simulink model "AFE_FV_RC_2L_Hacheur_4_Quadrants"  (R2013a)
settings: Solver=FixedStepDiscrete  SolverMode=SingleTasking  StartTime=0.0  StopTime=inf  FixedStep=Tpas  RelTol=1e-3
values from neighbouring files (symbols this model uses):
  Cbus = 300e-3    (= 0.3)    [AFE_FV_Params.m]
  Freq = 50    [AFE_FV_Params.m]
  hys = 100    [AFE_FV_Params.m]
  Iv = (Pv+Numdv(2)/Dendv(1))/Tsv    [AFE_FV_Params.m]
  Kac = 1/(Vac*sqrt(2/3))    [AFE_FV_Params.m]
  Lac = 8.1487e-04    (= 0.00081487)    [AFE_FV_Params.m]
  Pv = Numdv(1)/Dendv(1)    [AFE_FV_Params.m]
  Rch = 12    [AFE_FV_Params.m]
  Satv = 1500    [AFE_FV_Params.m]
  Tpas = 5e-5    (= 5e-05)    [AFE_FV_Params.m]
  Vac = 2000    [AFE_FV_Params.m]
undefined symbols (not defined in the file or in its folder): Rac
libraries: powerlib x30, simulink x8, powerlib_meascontrol x7
settings Model: Creator=LiberT  LastModifiedBy=Francis
settings DataIOCC: SignalLoggingSaveFormat=ModelDataLogs
settings OptimizationCC: ExpressionDepthLimit=2147483647
settings DebuggingCC: MultiTaskDSMMsg=warning  MultiTaskCondExecSysMsg=none  FcnCallInpInsideContextMsg=EnableAllAsWarning  StrictBusMsg=None
settings RTWCC: IncludeERTFirstTime=on

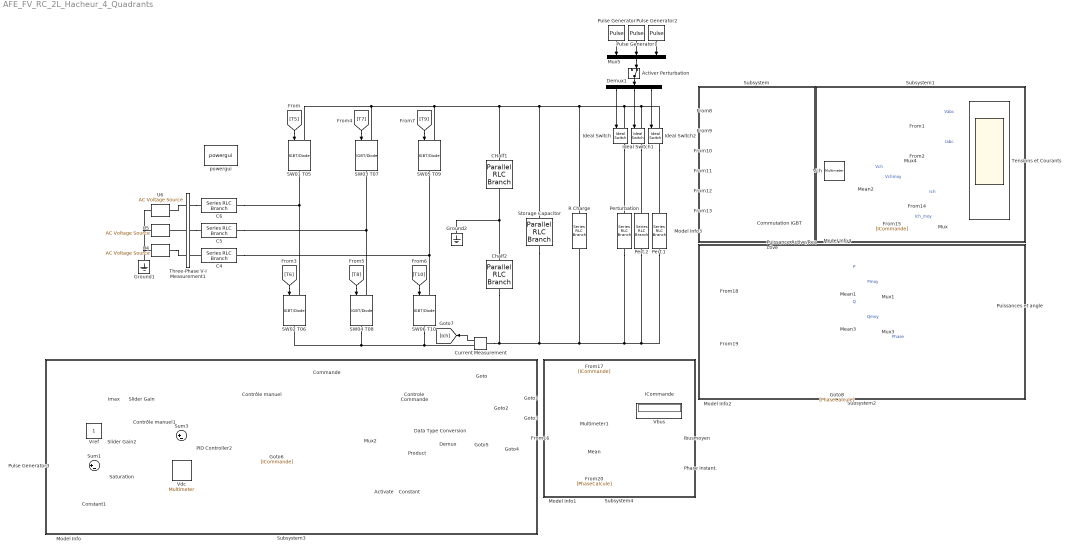
== system AFE_FV_RC_2L_Hacheur_4_Quadrants ==
  Activate : Constant  Value=0
  Activer Perturbation : ManualSwitch  CurrentSetting=0
  C4 : powerlib/Elements/Series RLC Branch  LConnTagsString=__new0  RConnTagsString=__new0  BranchType=L  Resistance=Rac  Inductance=Lac  SetiL0=off  InitialCurrent=0  Capacitance=300e-3  Setx0=off  InitialVoltage=0  Measurements=None
  C5 : powerlib/Elements/Series RLC Branch  LConnTagsString=__new0  RConnTagsString=__new0  BranchType=L  Resistance=Rac  Inductance=Lac  SetiL0=off  InitialCurrent=0  Capacitance=300e-3  Setx0=off  InitialVoltage=0  Measurements=None
  C6 : powerlib/Elements/Series RLC Branch  LConnTagsString=__new0  RConnTagsString=__new0  BranchType=L  Resistance=Rac  Inductance=Lac  SetiL0=off  InitialCurrent=0  Capacitance=300e-3  Setx0=off  InitialVoltage=0  Measurements=None
  CHalf1 : powerlib/Elements/Parallel RLC Branch  LConnTagsString=a  RConnTagsString=__new0  BranchType=C  Resistance=inf  Inductance=inf  SetiL0=off  InitialCurrent=0  Capacitance=.018  Setx0=off  InitialVoltage=2500  Measurements=Branch voltage
  Chalf2 : powerlib/Elements/Parallel RLC Branch  LConnTagsString=a  RConnTagsString=__new0  BranchType=C  Resistance=inf  Inductance=inf  SetiL0=off  InitialCurrent=0  Capacitance=.018  Setx0=off  InitialVoltage=2500  Measurements=Branch voltage
  Commande : Subsystem
  Commutation IGBT : Scope  NumInputPorts=6
      settings: TickLabels=on  TimeRange=0.04  YMin=-0.2~-0.2~-0.2~-0.2~-0.2~-0.2  YMax=1.2~1.2~1.2~1.2~1.2~1.2
  Constant : Constant  Value=[1 1 1 1 1 1]
  Constant1 : Constant  Value=6000
  Controle Commande : ManualSwitch
  Contrôle manuel : ManualSwitch  CurrentSetting=0
  Contrôle manuel1 : ManualSwitch  CurrentSetting=0
  Current Measurement : powerlib/Measurements/Current Measurement  PhasorSimulation=off  OutputType=Complex  PSBequivalent=0
  Data Type Conversion : DataTypeConversion  OutDataTypeStr=boolean
  Demux : Demux  Outputs=6
  Demux1 : Demux  Outputs=3
  Ground1 : powerlib/Elements/Ground  LConnTagsString=a
  Ground2 : powerlib/Elements/Ground  LConnTagsString=a
  "ICommande " : Display
  Ibusmoyen : Display
  Ideal Switch : powerlib/Power Electronics/Ideal Switch  Ron=0.001  Lon=0  IC=0  Rs=1e5  Cs=inf  Measurements=on
  Ideal Switch1 : powerlib/Power Electronics/Ideal Switch  Ron=0.001  Lon=0  IC=0  Rs=1e5  Cs=inf  Measurements=on
  Ideal Switch2 : powerlib/Power Electronics/Ideal Switch  Ron=0.001  Lon=0  IC=0  Rs=1e5  Cs=inf  Measurements=on
  Imax : Constant  Value=5000
  Mean{,1..3} (4 alike) : powerlib_meascontrol/Measurements/Mean  Freq=50  Vinit=0  Ts=Tpas
  Model Info : simulink/Model-Wide Utilities/Model Info  InitialBlockCM=None  BlockCM=None  Frame=on  DisplayStringWithTags=Commande  HorizontalTextAlignment=Center  LeftAlignmentValue=0.5  SourceBlockDiagram=AFE_FV_RC_2L_Hys  TagMaxNumber=20
  Model Info{1..4} (4 alike) : simulink/Model-Wide Utilities/Model Info  InitialBlockCM=None  BlockCM=None  Frame=on  DisplayStringWithTags=Résultats  HorizontalTextAlignment=Center  LeftAlignmentValue=0.5  SourceBlockDiagram=AFE_FV_RC_2L_Hys  TagMaxNumber=20
  Multimeter1 : powerlib/Measurements/Multimeter  PhasorSimulation=off  OutputType=Complex  sel=1  L=6  Gain=1  yselected={'Ub: Storage Capacitor'};  PSBOutputType=1  PSBequivalent=0  AxesSetting=[0,0.1,-100,100]  Display=0  SavedBlockNames=-11
  Mux{,1,3..4} (4 alike) : Mux  Inputs=2
  Mux2 : Mux  Inputs=6
  Mux5 : Mux  Inputs=3
  PID Controller2 : simulink/Continuous/PID Controller  Controller=PI  TimeDomain=Discrete-time  SampleTime=Tpas  IntegratorMethod=Forward Euler  FilterMethod=Forward Euler  Form=Parallel  P=Pv  I=Iv  D=0  N=100  InitialConditionSource=internal  InitialConditionForIntegrator=0  InitialConditionForFilter=0  ExternalReset=none  LimitOutput=on  UpperSaturationLimit=Satv  LowerSaturationLimit=-Satv  LinearizeAsGain=on  AntiWindupMode=clamping  Kb=1  TrackingMode=off  Kt=1  PParamMin=[]  PParamMax=[]  IParamMin=[]  IParamMax=[]  DParamMin=[]  DParamMax=[]  NParamMin=[]  NParamMax=[]  KbParamMin=[]  KbParamMax=[]  KtParamMin=[]  KtParamMax=[]  POutMin=[]  POutMax=[]  IOutMin=[]  IOutMax=[]  DOutMin=[]  DOutMax=[]  NOutMin=[]  NOutMax=[]  KbOutMin=[]  KbOutMax=[]  KtOutMin=[]  KtOutMax=[]  IntegratorOutMin=[]  IntegratorOutMax=[]  FilterOutMin=[]  FilterOutMax=[]  SumOutMin=[]  SumOutMax=[]  SumI1OutMin=[]  SumI1OutMax=[]  SumI2OutMin=[]  SumI2OutMax=[]  SumI3OutMin=[]  SumI3OutMax=[]  SumDOutMin=[]  SumDOutMax=[]  SaturationOutMin=[]  SaturationOutMax=[]  IntegratorContinuousStateAttributes=''  IntegratorStateMustResolveToSignalObject=off  IntegratorRTWStateStorageClass=Auto  FilterContinuousStateAttributes=''  FilterStateMustResolveToSignalObject=off  FilterRTWStateStorageClass=Auto
  Pert.1 : powerlib/Elements/Series RLC Branch  LConnTagsString=__new0  RConnTagsString=__new0  BranchType=R  Resistance=50  Inductance=0  SetiL0=off  InitialCurrent=0  Capacitance=inf  Setx0=off  InitialVoltage=0  Measurements=None
  Pert.2 : powerlib/Elements/Series RLC Branch  LConnTagsString=__new0  RConnTagsString=__new0  BranchType=R  Resistance=50  Inductance=0  SetiL0=off  InitialCurrent=0  Capacitance=inf  Setx0=off  InitialVoltage=0  Measurements=None
  Perturbation : powerlib/Elements/Series RLC Branch  LConnTagsString=__new0  RConnTagsString=__new0  BranchType=R  Resistance=50  Inductance=0  SetiL0=off  InitialCurrent=0  Capacitance=inf  Setx0=off  InitialVoltage=0  Measurements=None
  Phase instant. : Display
  Product : Product
  Puissance Active/Reactive : Subsystem
  Puissances et angle : Scope  NumInputPorts=3
      settings: TickLabels=on  TimeRange=0.04  YMin=-3.1e+06~-400000~-200  YMax=-2.1e+06~350000~200  SaveName=ScopeData2
  Pulse Generator : DiscretePulseGenerator  Period=floor((1/Tpas)/2)  PulseWidth=floor((1/Tpas)/4)  SampleTime=Tpas
  Pulse Generator1 : DiscretePulseGenerator  Period=floor((1/Tpas)/3)  PulseWidth=floor((1/Tpas)/6)  SampleTime=Tpas
  Pulse Generator2 : DiscretePulseGenerator  Period=floor((1/Tpas))  PulseWidth=floor((1/Tpas)/2)  SampleTime=Tpas
  Pulse Generator3 : DiscretePulseGenerator  Amplitude=12000  Period=floor(.2/Tpas)  PulseWidth=floor(.2/2/Tpas)  SampleTime=Tpas
  R Charge : powerlib/Elements/Series RLC Branch  LConnTagsString=__new0  RConnTagsString=__new0  BranchType=R  Resistance=Rch  Inductance=0  SetiL0=off  InitialCurrent=0  Capacitance=inf  Setx0=off  InitialVoltage=0  Measurements=None
  SW01 T05 : powerlib/Power Electronics/IGBT//Diode  Ron=1e-3  Rs=1e5  Cs=Tpas  Measurements=off
  SW02 T06 : powerlib/Power Electronics/IGBT//Diode  Ron=1e-3  Rs=1e5  Cs=Tpas  Measurements=off
  SW03 T07 : powerlib/Power Electronics/IGBT//Diode  Ron=1e-3  Rs=1e5  Cs=Tpas  Measurements=off
  SW04 T08 : powerlib/Power Electronics/IGBT//Diode  Ron=1e-3  Rs=1e5  Cs=Tpas  Measurements=off
  SW05 T09 : powerlib/Power Electronics/IGBT//Diode  Ron=1e-3  Rs=1e5  Cs=Tpas  Measurements=off
  SW06 T10 : powerlib/Power Electronics/IGBT//Diode  Ron=1e-3  Rs=1e5  Cs=Tpas  Measurements=off
  Saturation : Saturate  UpperLimit=5100  LowerLimit=5000
  Slider Gain : simulink/Math Operations/Slider Gain  low=0  gain=0.22  high=1
  Slider Gain2 : simulink/Math Operations/Slider Gain  low=0  gain=5000  high=6000
  Storage Capacitor : powerlib/Elements/Parallel RLC Branch  LConnTagsString=a  RConnTagsString=__new0  BranchType=C  Resistance=inf  Inductance=inf  SetiL0=off  InitialCurrent=0  Capacitance=Cbus  Setx0=on  InitialVoltage=Vdc  Measurements=Branch voltage
  Subsystem : Subsystem
      mask Display: disp('')
  Subsystem1 : Subsystem
      mask Display: disp('')
  Subsystem2 : Subsystem
      mask Display: disp('')
  Subsystem3 : Subsystem
      mask Display: disp('')
  Subsystem4 : Subsystem
      mask Display: disp('')
  Sum1 : Sum  Inputs=|+-
  Sum3 : Sum  Inputs=|+-
  Tensions et Courants : Scope  NumInputPorts=4
      settings: TickLabels=on  ShowLegends=on  TimeRange=0.04  YMin=-1750~-2000~4900~-2000  YMax=1750~2000~5150~2000
  Three-Phase V-I Measurement1 : powerlib/Measurements/Three-Phase V-I Measurement  VoltageMeasurement=phase-to-ground  SetLabelV=on  LabelV=Vabc  Vpu=off  VpuLL=off  CurrentMeasurement=yes  SetLabelI=on  LabelI=Iabc  Ipu=off  Pbase=100e6  Vbase=500e3  OutputType=Complex  PhasorSimulation=off  PSBequivalent=0
  U4 : powerlib/Electrical Sources/AC Voltage Source  Amplitude=Vac*sqrt(2/3)  Phase=120  Frequency=Freq  SampleTime=Tpas  Measurements=Voltage
  U5 : powerlib/Electrical Sources/AC Voltage Source  Amplitude=Vac*sqrt(2/3)  Phase=-120  Frequency=Freq  SampleTime=Tpas  Measurements=Voltage
  U6 : powerlib/Electrical Sources/AC Voltage Source  Amplitude=Vac*sqrt(2/3)  Phase=0  Frequency=Freq  SampleTime=Tpas  Measurements=Voltage
  Vbus : Display
  Vch : powerlib/Measurements/Multimeter  PhasorSimulation=off  OutputType=Complex  sel=1  L=6  Gain=1  yselected={'Ub: Storage Capacitor'};  PSBOutputType=1  PSBequivalent=0  AxesSetting=[0,0.1,-100,100]  Display=0  SavedBlockNames=-11
  Vdc : powerlib/Measurements/Multimeter  PhasorSimulation=off  OutputType=Complex  sel=1  L=6  Gain=1  yselected={'Ub: Storage Capacitor'};  PSBOutputType=1  PSBequivalent=0  AxesSetting=[0,0.1,-100,100]  Display=0  SavedBlockNames=-11
  Vref : Constant  SampleTime=Tpas
  powergui : powerlib/powergui  Priority=1  SimulationMode=Discrete  SolverType=Tustin  SampleTime=Tpas  frequency=60  SPID=off  DisableSnubberDevices=off  DisableRonSwitches=off  DisableVfSwitches=off  SwTol=0  Interpol=off  DisplayEquations=off  frequencyindice=50  Pbase=100e6  ErrMax=1e-4  Iterations=50  UnitsV=kV  UnitsW=MW  FunctionMessages=off  echomessages=off  HookPort=off  EnableUseOfTLC=off  x0status=blocks  RestoreLinks=warning  ResistiveCurrentMeasurement=off  Frange=[0:2:500]  Ylog=off  Xlog=on  ShowGrid=off  save=off  variable=ZData  structure=ScopeData1  ZoomFFT=off  StartTime=18  cycles=100  DisplayStyle=1  fundamental=50  FreqAxis=off  MaxFrequency=2000  frequencyindicesteady=1  RmsSteady=1  display=off  Ts=0  methode=off
  wires:
  [T5] -> SW01 T05/1
  Current Measurement/1 -> [Ich]
  [T7] -> SW03 T07/1
  [T9] -> SW05 T09/1
  [T10] -> SW06 T10/1
  [T8] -> SW04 T08/1
  [T6] -> SW02 T06/1
  [T5] -> Commutation IGBT/1
  [T6] -> Commutation IGBT/2
  [T7] -> Commutation IGBT/3
  [T8] -> Commutation IGBT/4
  [T9] -> Commutation IGBT/5
  [T10] -> Commutation IGBT/6
  [Vabc] -> Tensions et Courants/1  "Vabc"
  [Iabc] -> Tensions et Courants/2  "Iabc"
  Imax/1 -> Slider Gain/1
  [Ich] -> Mux/1  "Ich"
  [ICommande] -> Mux/2  "Ich_moy"
  Mux/1 -> Tensions et Courants/4
  Mean/1 -> Ibusmoyen/1
  Multimeter1/1 -> Vbus/1
  [Ich] -> Mean/1
  [ICommande] -> "ICommande "/1
  Vdc/1 -> Sum3/2
  Vref/1 -> Slider Gain2/1
  Sum3/1 -> PID Controller2/1
  Constant/1 -> Product/2
  Activate/1 -> Product/1
  Commande/1(T5) -> Mux2/1
  Commande/2(T6) -> Mux2/2
  Commande/3(T7) -> Mux2/3
  Commande/4(T8) -> Mux2/4
  Commande/5(T9) -> Mux2/5
  Commande/6(T10) -> Mux2/6
  Controle Commande/1 -> Demux/1
  Mux2/1 -> Controle Commande/1
  Demux/1 -> [T5]
  Demux/2 -> [T6]
  Demux/3 -> [T7]
  Demux/4 -> [T8]
  Demux/5 -> [T9]
  Demux/6 -> [T10]
  [Vabc] -> Puissance Active/Reactive/1(Vabc)
  [Iabc] -> Puissance Active/Reactive/2(Iabc)
  Puissance Active/Reactive/1(P) -> Mux1/1, Mean1/1  "P"
  Puissance Active/Reactive/2(Q) -> Mean3/1, Mux3/1  "Q"
  Puissance Active/Reactive/3(PhC) -> Puissances et angle/3, [PhaseCalcule]  "Phase"
  Mean1/1 -> Mux1/2  "Pmoy"
  Mux1/1 -> Puissances et angle/1
  Mean3/1 -> Mux3/2  "Qmoy"
  Mux3/1 -> Puissances et angle/2
  Mux4/1 -> Tensions et Courants/3
  Vch/1 -> Mux4/1, Mean2/1  "Vch"
  Mean2/1 -> Mux4/2  "Vchmoy"
  Demux1/1 -> Ideal Switch/1
  Demux1/2 -> Ideal Switch1/1
  Demux1/3 -> Ideal Switch2/1
  Pulse Generator/1 -> Mux5/1
  Pulse Generator1/1 -> Mux5/2
  Pulse Generator2/1 -> Mux5/3
  Activer Perturbation/1 -> Demux1/1
  Mux5/1 -> Activer Perturbation/2
  [PhaseCalcule] -> Phase instant./1
  PID Controller2/1 -> Contrôle manuel/2
  Slider Gain/1 -> Contrôle manuel/1
  Contrôle manuel/1 -> Commande/1(In1), [ICommande]
  Data Type Conversion/1 -> Controle Commande/2
  Product/1 -> Data Type Conversion/1
  Sum1/1 -> Saturation/1
  Pulse Generator3/1 -> Sum1/1
  Constant1/1 -> Sum1/2
  Contrôle manuel1/1 -> Sum3/1
  Slider Gain2/1 -> Contrôle manuel1/1
  Saturation/1 -> Contrôle manuel1/2
  connections:
  Current Measurement/RConn1 -- SW06 T10/RConn1 -- SW04 T08/RConn1 -- SW02 T06/RConn1
  SW01 T05/LConn1 -- Ideal Switch1/LConn1 -- Ideal Switch2/LConn1 -- Ideal Switch/LConn1 -- R Charge/LConn1 -- Storage Capacitor/LConn1 -- CHalf1/LConn1 -- SW05 T09/LConn1 -- SW03 T07/LConn1
  SW02 T06/LConn1 -- C6/LConn1 -- SW01 T05/RConn1
  SW06 T10/LConn1 -- C4/LConn1 -- SW05 T09/RConn1
  SW04 T08/LConn1 -- C5/LConn1 -- SW03 T07/RConn1
  Three-Phase V-I Measurement1/LConn1 -- C6/RConn1
  Three-Phase V-I Measurement1/RConn1 -- U6/RConn1
  Three-Phase V-I Measurement1/RConn2 -- U5/RConn1
  Three-Phase V-I Measurement1/LConn2 -- C5/RConn1
  C4/RConn1 -- Three-Phase V-I Measurement1/LConn3
  U4/RConn1 -- Three-Phase V-I Measurement1/RConn3
  Storage Capacitor/RConn1 -- Chalf2/RConn1 -- Current Measurement/LConn1 -- Pert.2/RConn1 -- Pert.1/RConn1 -- Perturbation/RConn1 -- R Charge/RConn1
  U4/LConn1 -- U6/LConn1 -- U5/LConn1 -- Ground1/LConn1
  Ideal Switch/RConn1 -- Perturbation/LConn1
  Ideal Switch1/RConn1 -- Pert.2/LConn1
  Ideal Switch2/RConn1 -- Pert.1/LConn1
  Chalf2/LConn1 -- Ground2/LConn1 -- CHalf1/RConn1

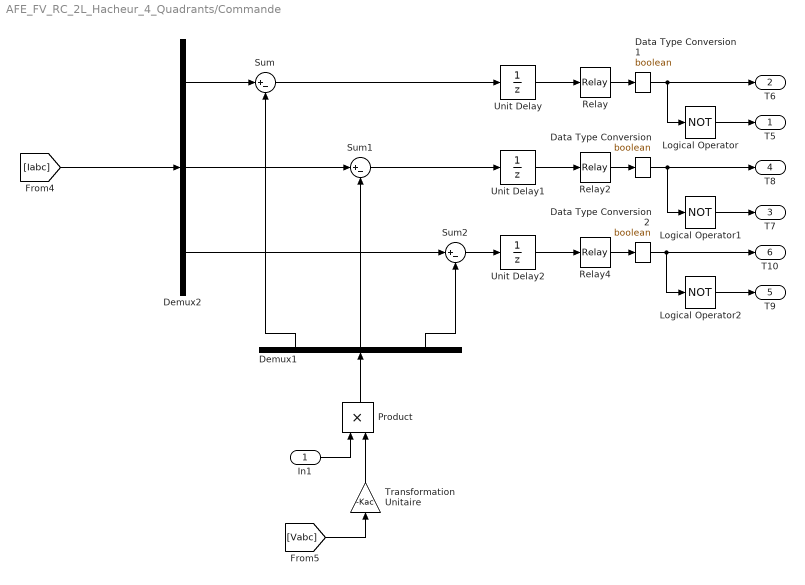
== system AFE_FV_RC_2L_Hacheur_4_Quadrants/Commande ==
  In1 : Inport
  Data Type Conversion : DataTypeConversion  OutDataTypeStr=boolean
  Data Type Conversion1 : DataTypeConversion  OutDataTypeStr=boolean
  Data Type Conversion2 : DataTypeConversion  OutDataTypeStr=boolean
  Demux1 : Demux  Outputs=3
  Demux2 : Demux  Outputs=3
  Logical Operator : Logic  Operator=NOT  AllPortsSameDT=off
  Logical Operator1 : Logic  Operator=NOT  AllPortsSameDT=off
  Logical Operator2 : Logic  Operator=NOT  AllPortsSameDT=off
  Product : Product
  Relay : Relay  OnSwitchValue=hys  OffSwitchValue=-hys
  Relay2 : Relay  OnSwitchValue=hys  OffSwitchValue=-hys
  Relay4 : Relay  OnSwitchValue=hys  OffSwitchValue=-hys
  Sum : Sum  Inputs=|+-
  Sum1 : Sum  Inputs=|+-
  Sum2 : Sum  Inputs=|+-
  Transformation Unitaire : Gain  Gain=-Kac
  Unit Delay : UnitDelay  SampleTime=-1
  Unit Delay1 : UnitDelay  SampleTime=-1
  Unit Delay2 : UnitDelay  SampleTime=-1
  T5 : Outport
  T6 : Outport  Port=2
  T7 : Outport  Port=3
  T8 : Outport  Port=4
  T9 : Outport  Port=5
  T10 : Outport  Port=6
  wires:
  Demux2/1 -> Sum/1
  Demux2/2 -> Sum1/1
  Demux2/3 -> Sum2/1
  Sum/1 -> Unit Delay/1
  Sum1/1 -> Unit Delay1/1
  Sum2/1 -> Unit Delay2/1
  Unit Delay/1 -> Relay/1
  Unit Delay1/1 -> Relay2/1
  Unit Delay2/1 -> Relay4/1
  Logical Operator/1 -> T5/1
  Logical Operator1/1 -> T7/1
  Logical Operator2/1 -> T9/1
  Relay/1 -> Data Type Conversion1/1
  Relay2/1 -> Data Type Conversion/1
  Relay4/1 -> Data Type Conversion2/1
  [Iabc] -> Demux2/1
  [Vabc] -> Transformation Unitaire/1
  Demux1/1 -> Sum/2
  Demux1/2 -> Sum1/2
  Demux1/3 -> Sum2/2
  Data Type Conversion/1 -> T8/1, Logical Operator1/1
  Data Type Conversion1/1 -> T6/1, Logical Operator/1
  Data Type Conversion2/1 -> T10/1, Logical Operator2/1
  Transformation Unitaire/1 -> Product/2
  In1/1 -> Product/1
  Product/1 -> Demux1/1

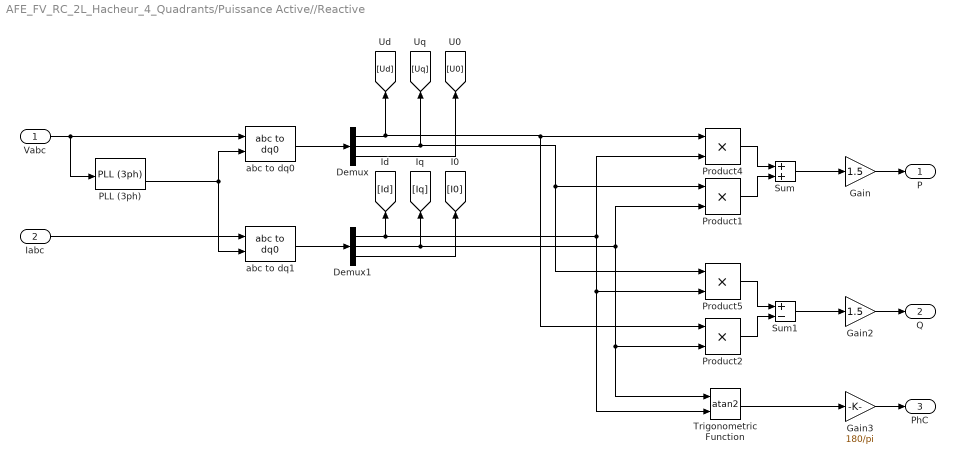
== system AFE_FV_RC_2L_Hacheur_4_Quadrants/Puissance Active//Reactive ==
  Vabc : Inport
  Iabc : Inport  Port=2
  Demux : Demux  Outputs=3
  Demux1 : Demux  Outputs=3
  Gain : Gain  Gain=1.5
  Gain2 : Gain  Gain=1.5
  Gain3 : Gain  Gain=180/pi
  PLL (3ph) : powerlib_meascontrol/PLL/PLL (3ph)  Fmin=49  Par_Init=[0, 50]  ParK=[180, 3200, 1]  TcD=1e-4  MaxRateChangeFreq=6  FilterCutOffFreq=25  Ts=Tpas  AGC=on
  Product{1..2,4..5} (4 alike) : Product
  Sum : Sum
  Sum1 : Sum  Inputs=+-
  Trigonometric Function : Trigonometry  Operator=atan2
  abc to dq0 : powerlib_meascontrol/Transformations/abc to dq0  Alignment=90 degrees behind phase A axis
  abc to dq1 : powerlib_meascontrol/Transformations/abc to dq0  Alignment=90 degrees behind phase A axis
  P : Outport
  Q : Outport  Port=2
  PhC : Outport  Port=3
  wires:
  Vabc/1 -> PLL (3ph)/1, abc to dq0/1
  abc to dq0/1 -> Demux/1
  abc to dq1/1 -> Demux1/1
  Product2/1 -> Sum1/2
  Sum1/1 -> Gain2/1
  Demux/3 -> [U0]
  Demux/2 -> Product5/1, Product1/1, [Uq]
  Demux/1 -> Product2/1, Product4/1, [Ud]
  Demux1/2 -> [Iq], Trigonometric Function/1, Product2/2, Product1/2
  Product5/1 -> Sum1/1
  Gain2/1 -> Q/1
  Trigonometric Function/1 -> Gain3/1
  Gain3/1 -> PhC/1
  Product4/1 -> Sum/1
  Product1/1 -> Sum/2
  Sum/1 -> Gain/1
  Gain/1 -> P/1
  Demux1/1 -> [Id], Trigonometric Function/2, Product5/2, Product4/2
  Demux1/3 -> [I0]
  PLL (3ph)/2 -> abc to dq1/2, abc to dq0/2
  Iabc/1 -> abc to dq1/1

== system AFE_FV_RC_2L_Hacheur_4_Quadrants/Subsystem ==

== system AFE_FV_RC_2L_Hacheur_4_Quadrants/Subsystem1 ==

== system AFE_FV_RC_2L_Hacheur_4_Quadrants/Subsystem2 ==

== system AFE_FV_RC_2L_Hacheur_4_Quadrants/Subsystem3 ==

== system AFE_FV_RC_2L_Hacheur_4_Quadrants/Subsystem4 ==
